simulink library "House_OneNodeModel"  (R2016b)
settings: Solver=ode45  StartTime=0.0  StopTime=10.0  RelTol=1e-3  EnableMultiTasking=on
libraries: carnot x12
settings Model: Creator=lena.frank  LastModifiedBy=drhf
settings DataIOCC: LimitDataPoints=on  SaveFormat=Array  SignalLoggingSaveFormat=ModelDataLogs
settings OptimizationCC: ExpressionDepthLimit=2147483647  LifeSpan=inf
settings DebuggingCC: UnderspecifiedInitializationDetection=Classic  MergeDetectMultiDrivingBlocksExec=none  SolverPrmCheckMsg=warning  FcnCallInpInsideContextMsg=warning  StateNameClashWarn=warning  SFUnexpectedBacktrackingDiag=warning  SFNoUnconditionalDefaultTransitionDiag=warning  SFExecutionAtInitializationDiag=none
settings HardwareCC: ProdBitPerPointer=32  ProdBitPerSizeT=32  ProdBitPerPtrDiffT=32  ProdLargestAtomicFloat=None  ProdIntDivRoundTo=Undefined  ProdEndianess=Unspecified  ProdWordSize=32  ProdHWDeviceType=32-bit Generic
settings ModelReferenceCC: PropagateSignalLabelsOutOfModel=off
settings GRTTargetCC: TargetLangStandard=C89/C90 (ANSI)  GeneratePreprocessorConditionals=Disable all  CombineOutputUpdateFcns=off  GRTInterface=on
settings ConfigComp: CovMetricSettings=dw  CovHtmlReporting=on  CovSaveCumulativeToWorkspaceVar=on  CovSaveSingleToWorkspaceVar=on  CovExternalEMLEnable=off

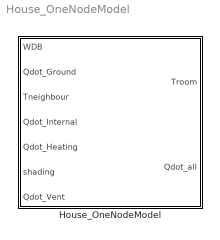
== system House_OneNodeModel ==
  House_OneNodeModel : Subsystem  mask(House One Node Model){Ahabit=120, Hroom=2.5, tini=20, UAout=200, mc=10e3*2000, UAin=0, dtroom=inf, AziWin=[0 90 180 270], Awin=[1 1 1 1], Uwin=[1 1 1 1], Gwin=[0.6 0.6 0.6 0.6]}
      mask prompts: Ahabit "living surface in m²"; Hroom "height of rooms in m"; tini "initial temperature"; UAout "heat loss of walls and roof in W/K"; mc "total thermal capacity in J/K"; UAin "heat transfer to neighbour in W/K"; dtroom "LIMITED TEMPERATURE CHANGE in K (standard value = 'inf')"; AziWin "orientation of 4 windows (south 0, east -90,west 90)"; Awin "surface of 4 windows in m² (vector)"; Uwin "heat loss coefficient 4 windows in W/m²/K [vector]"; Gwin "light transmittance 4 windows (0..1) * (1 - frame_part) [vector]"
      mask help:
      | Simple model of 1-node room or house. The differential equation is solved:
      | (m*c)house * dT/dt = solar_gain + internal_gain + heating_power - losses_to_ambient - losses_to_neighbour_room
      | All powers on the right hand side are in W !
      | The heating_power is generated by a radiator or floor heating system.
      | A usual value for the internal_gain is (2.3 W/m² * Ahabit).
      | The windows have a shading for solar radiation (standard value is 1):
      | solar gain = Solar_Radiation_on_window * WindowSurface* light_transmittance * shading_factor
      |
      | LIMITED TEMPERATURE CHANGE: If you want to calculate idealized heating behaviour. 0 K means that the room temperature is fixed, the power balace is the theoretical heating demand (see example_House_Ideal.mdl).
      mask init:
      | invmc = 1/mc;
      | Gwin = max(0,min(1,Gwin));
      mask Help: web(fullfile(path_carnot('help'),'Simple_House.html'),'-helpbrowser')
      mask Display: plot(0,-15,80,100,[30,30,60,60,30],[20,50,50,20,20],[47,47,56,56,47],[40,30,30,40,40],[42,42,34,34],[20,40,40,20],[62,45,28],[48,70,48])

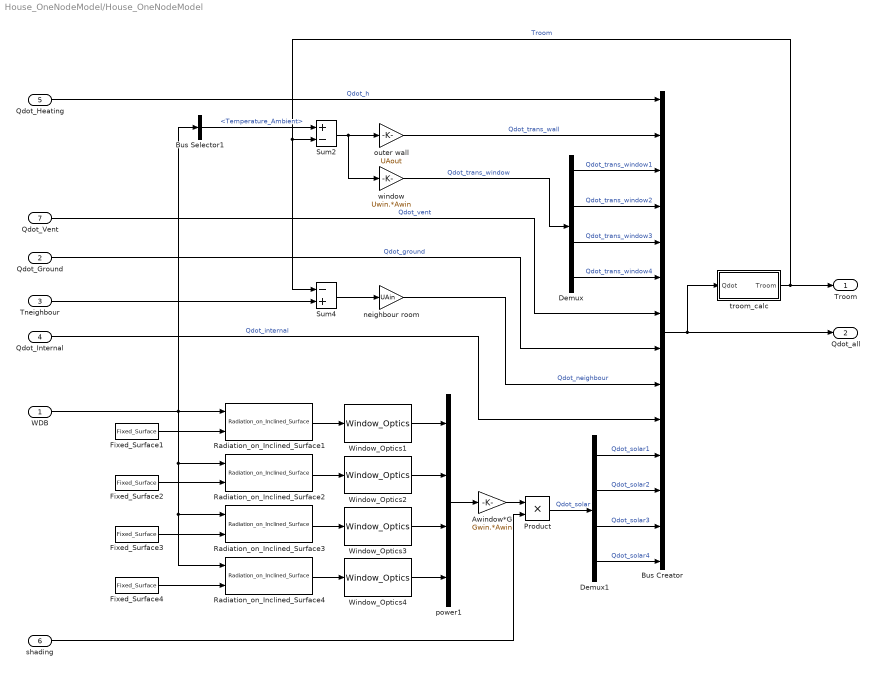
== system House_OneNodeModel/House_OneNodeModel ==
  WDB : Inport
  Qdot_Ground : Inport  Port=2
  Tneighbour : Inport  Port=3
  Qdot_Internal : Inport  Port=4
  Qdot_Heating : Inport  Port=5
  shading : Inport  Port=6
  Qdot_Vent : Inport  Port=7
  Awindow*G : Gain  Gain=Gwin.*Awin  SaturateOnIntegerOverflow=on  OutDataTypeStr=Inherit: Same as input  ParamDataTypeStr=Inherit: Same as input
  Bus Creator : BusCreator  Inputs=14
  Bus Selector1 : BusSelector  OutputSignals=Temperature_Ambient
  Demux : Demux
  Demux1 : Demux
  Fixed_Surface1 : carnot/Weather/Fixed_Surface  colangle=90  colazi=AziWin(1)  colrot=0
  Fixed_Surface2 : carnot/Weather/Fixed_Surface  colangle=90  colazi=AziWin(2)  colrot=0
  Fixed_Surface3 : carnot/Weather/Fixed_Surface  colangle=90  colazi=AziWin(3)  colrot=0
  Fixed_Surface4 : carnot/Weather/Fixed_Surface  colangle=90  colazi=AziWin(4)  colrot=0
  Product : Product  RndMeth=Zero
  Radiation_on_Inclined_Surface{1..4} (4 alike) : carnot/Weather/Radiation_on_Inclined_Surface  sky=Perez 1990  reflect=0.2
  Sum2 : Sum  Inputs=+-  SaturateOnIntegerOverflow=on  InputSameDT=on  OutDataTypeStr=Inherit: Same as first input
  Sum4 : Sum  Inputs=-+  SaturateOnIntegerOverflow=on  InputSameDT=on  OutDataTypeStr=Inherit: Same as first input
  Window_Optics{1..4} (4 alike) : carnot/Load/Houses/wall_floor/Window_Optics
  neighbour room : Gain  Gain=UAin  SaturateOnIntegerOverflow=on  OutDataTypeStr=Inherit: Same as input  ParamDataTypeStr=Inherit: Same as input
  outer wall : Gain  Gain=UAout  SaturateOnIntegerOverflow=on  OutDataTypeStr=Inherit: Same as input  ParamDataTypeStr=Inherit: Same as input
  power1 : Mux
  troom_calc : Subsystem
  window : Gain  Gain=Uwin.*Awin  SaturateOnIntegerOverflow=on  OutDataTypeStr=Inherit: Same as input  ParamDataTypeStr=Inherit: Same as input
  Troom : Outport
  Qdot_all : Outport  Port=2
  wires:
  Qdot_Internal/1 -> Bus Creator/10  "Qdot_internal"
  Demux/4 -> Bus Creator/6  "Qdot_trans_window4"
  Demux/3 -> Bus Creator/5  "Qdot_trans_window3"
  Demux/2 -> Bus Creator/4  "Qdot_trans_window2"
  Demux1/3 -> Bus Creator/13  "Qdot_solar3"
  Demux1/2 -> Bus Creator/12  "Qdot_solar2"
  Demux1/1 -> Bus Creator/11  "Qdot_solar1"
  Demux1/4 -> Bus Creator/14  "Qdot_solar4"
  window/1 -> Demux/1  "Qdot_trans_window"
  troom_calc/1(Troom) -> Sum2/2, Sum4/1, Troom/1  "Troom"
  Radiation_on_Inclined_Surface4/1 -> Window_Optics4/1
  Fixed_Surface4/1 -> Radiation_on_Inclined_Surface4/2
  Radiation_on_Inclined_Surface3/1 -> Window_Optics3/1
  Fixed_Surface3/1 -> Radiation_on_Inclined_Surface3/2
  Radiation_on_Inclined_Surface2/1 -> Window_Optics2/1
  Fixed_Surface2/1 -> Radiation_on_Inclined_Surface2/2
  power1/1 -> Awindow*G/1
  Radiation_on_Inclined_Surface1/1 -> Window_Optics1/1
  Fixed_Surface1/1 -> Radiation_on_Inclined_Surface1/2
  neighbour room/1 -> Bus Creator/9  "Qdot_neighbour"
  Demux/1 -> Bus Creator/3  "Qdot_trans_window1"
  Sum4/1 -> neighbour room/1
  Qdot_Ground/1 -> Bus Creator/8  "Qdot_ground"
  Bus Creator/1 -> Qdot_all/1, troom_calc/1(Qdot)
  WDB/1 -> Bus Selector1/1, Radiation_on_Inclined_Surface1/1, Radiation_on_Inclined_Surface2/1, Radiation_on_Inclined_Surface4/1, Radiation_on_Inclined_Surface3/1
  Bus Selector1/1 -> Sum2/1  "<Temperature_Ambient>"
  outer wall/1 -> Bus Creator/2  "Qdot_trans_wall"
  Sum2/1 -> window/1, outer wall/1
  Product/1 -> Demux1/1  "Qdot_solar"
  Window_Optics1/1 -> power1/1
  Window_Optics2/1 -> power1/2
  Window_Optics3/1 -> power1/3
  Window_Optics4/1 -> power1/4
  Qdot_Heating/1 -> Bus Creator/1  "Qdot_h"
  Awindow*G/1 -> Product/1
  shading/1 -> Product/2
  Qdot_Vent/1 -> Bus Creator/7  "Qdot_vent"
  Tneighbour/1 -> Sum4/2

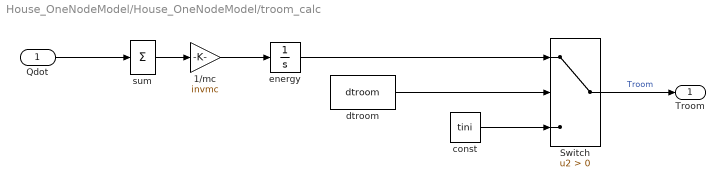
== system House_OneNodeModel/House_OneNodeModel/troom_calc ==
  Qdot : Inport
  1/mc : Gain  Gain=invmc  SaturateOnIntegerOverflow=on  OutDataTypeStr=Inherit: Same as input  ParamDataTypeStr=Inherit: Same as input
  Switch : Switch  Criteria=u2 > Threshold
  const : Constant  Value=tini
  dtroom : Constant  Value=dtroom
  energy : Integrator  InitialCondition=tini  LimitOutput=on  UpperSaturationLimit=tini+max(0.01,dtroom)  LowerSaturationLimit=tini-max(0.01,dtroom)
  sum : Sum  Inputs=1  SaturateOnIntegerOverflow=on  InputSameDT=on  OutDataTypeStr=Inherit: Same as first input
  Troom : Outport
  wires:
  const/1 -> Switch/3
  sum/1 -> 1/mc/1
  1/mc/1 -> energy/1
  energy/1 -> Switch/1
  Switch/1 -> Troom/1  "Troom"
  dtroom/1 -> Switch/2
  Qdot/1 -> sum/1
